simulink model "questao1lcsd2"  (R2026a)
settings: Solver=VariableStepAuto
libraries: dspstat3 x1
settings Model: Creator=shumy  LastModifiedBy=shumy

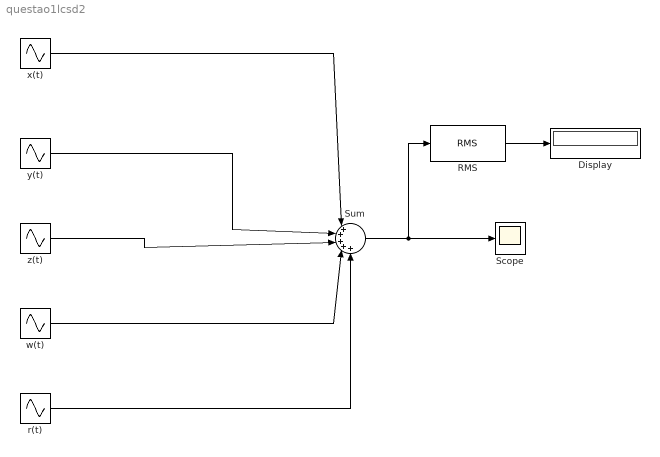
== system questao1lcsd2 ==
  Display : Display
  RMS : dspstat3/RMS  run=off  directionMode=Each column  dimension=1  InputProcessing=Columns as channels (frame based)  reset_popup=None
  Scope : Scope
      settings: ActiveDisplayYMinimum=-4.6328830327869  ActiveDisplayYMaximum=4.6413252042280337
  Sum : Sum  Inputs=|+++++
  r(t) : Sin  Amplitude=4/9  Frequency=18  SampleTime=0
  w(t) : Sin  Amplitude=4/7  Frequency=14  SampleTime=0
  x(t) : Sin  Amplitude=4  Frequency=2  SampleTime=0
  y(t) : Sin  Amplitude=4/3  Frequency=6  SampleTime=0
  z(t) : Sin  Amplitude=4/5  Frequency=10  SampleTime=0
  wires:
  x(t)/1 -> Sum/1
  y(t)/1 -> Sum/2
  z(t)/1 -> Sum/3
  w(t)/1 -> Sum/4
  r(t)/1 -> Sum/5
  Sum/1 -> RMS/1, Scope/1
  RMS/1 -> Display/1
